simulink model "after_regulation"  (R2018a)
settings: Solver=VariableStepAuto  StartTime=0.0  StopTime=10.0  RelTol=1e-3
undefined symbols (not defined in the file or in its folder): sigbuilder_block
libraries: fuzblock x1
settings Model: Creator=root  LastModifiedBy=root

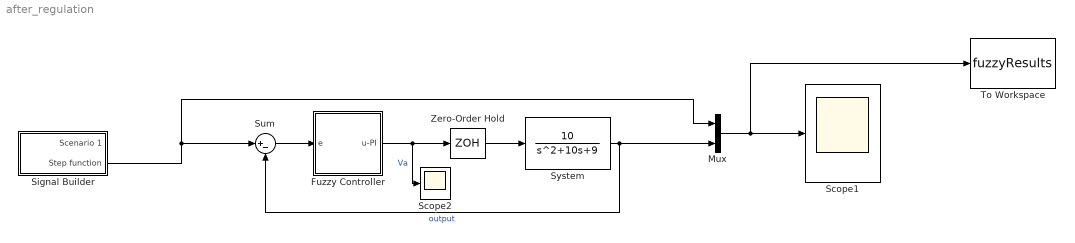
== system after_regulation ==
  Fuzzy Controller : Subsystem
  Mux : Mux  Inputs=2
  Scope1 : Scope
  Scope2 : Scope
  Signal Builder : Subsystem  Tag=STV Subsys  LoadFcn=sigbuilder_block('load');  StartFcn=sigbuilder_block('start');  StopFcn=sigbuilder_block('stop');  ClipboardFcn=sigbuilder_block('clipboard');  mask(Sigbuilder block){tuvar=[0:10]}
      mask help: Simulink:masks:SigbuilderBlock_MD
      mask init:
      | if ~strcmp(get_param(bdroot(gcbh),'SimulationStatus'),'stopped') tuvar = sigbuilder_block('maskInit'); end
      settings: CopyFcn=sigbuilder_block('copy');  DeleteFcn=sigbuilder_block('delete');  ModelCloseFcn=sigbuilder_block('modelClose');  PreSaveFcn=sigbuilder_block('preSave');  PauseFcn=sigbuilder_block('pause');  ContinueFcn=sigbuilder_block('continue');  NameChangeFcn=sigbuilder_block('namechange');  OpenFcn=sigbuilder_block('open',[225 75 550.5 393.75 ]);  CloseFcn=sigbuilder_block('close');
      mask Display: plot(0, 0, 100, 100,[2, 2, 32, 32, 2], [68, 8, 8, 68, 68],[32, 2], [38, 38], [32, 19, 2],[53, 60, 44], [32, 17, 17, 2],[16, 16, 31, 31]);txt = getActiveGroup(gcbh);text(2, 100, txt,'verticalAlignment', 'top');
  Sum : Sum  Inputs=|+-
  System : TransferFcn  Numerator=10  Denominator=[1 10 9]
  To Workspace : ToWorkspace  VariableName=fuzzyResults  SaveFormat=Timeseries  SampleTime=-1
  Zero-Order Hold : ZeroOrderHold  SampleTime=0.01
  wires:
  Zero-Order Hold/1 -> System/1
  System/1 -> Mux/2, Sum/2  "output"
  Fuzzy Controller/1(u-PI) -> Scope2/1, Zero-Order Hold/1  "Va"
  Signal Builder/2(Step function) -> Mux/1, Sum/1
  Sum/1 -> Fuzzy Controller/1(e)
  Mux/1 -> To Workspace/1, Scope1/1

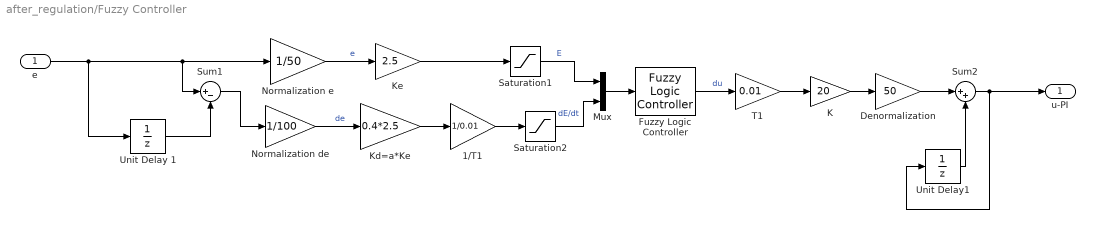
== system after_regulation/Fuzzy Controller ==
  e : Inport
  1/T1 : Gain  Gain=1/0.01
  Denormalization : Gain  Gain=50
  Fuzzy Logic Controller : fuzblock/Fuzzy Logic  Controller  FIS='satellite_8885'  OutputSampleNumber=101  DataType=single  FuzzifiedInputs=off  RuleFiringStrengths=off  RuleOutputs=off  AggregatedOutputs=off  SimulateUsing=Interpreted execution  OutOfRangeInputValueMessage=warning  NoRuleFiredMessage=warning  EmptyOutputFuzzySetMessage=warning
  K : Gain  Gain=20
  Kd=a*Ke : Gain  Gain=0.4*2.5
  Ke : Gain  Gain=2.5
  Mux : Mux  Inputs=2
  Normalization de : Gain  Gain=1/100
  Normalization e : Gain  Gain=1/50
  Saturation1 : Saturate  UpperLimit=1  LowerLimit=-1
  Saturation2 : Saturate  UpperLimit=1  LowerLimit=-1
  Sum1 : Sum  Inputs=|+-
  Sum2 : Sum  Inputs=|++
  T1 : Gain  Gain=0.01
  Unit Delay 1 : UnitDelay  SampleTime=-1
  Unit Delay1 : UnitDelay  SampleTime=-1
  u-PI : Outport
  wires:
  Normalization e/1 -> Ke/1  "e"
  Normalization de/1 -> Kd=a*Ke/1  "de"
  Saturation2/1 -> Mux/2  "dE/dt"
  e/1 -> Unit Delay 1/1, Sum1/1, Normalization e/1
  Unit Delay 1/1 -> Sum1/2
  Sum2/1 -> Unit Delay1/1, u-PI/1
  Saturation1/1 -> Mux/1  "E"
  Unit Delay1/1 -> Sum2/2
  Kd=a*Ke/1 -> 1/T1/1
  K/1 -> Denormalization/1
  Denormalization/1 -> Sum2/1
  Sum1/1 -> Normalization de/1
  Ke/1 -> Saturation1/1
  1/T1/1 -> Saturation2/1
  Mux/1 -> Fuzzy Logic Controller/1
  T1/1 -> K/1
  Fuzzy Logic Controller/1 -> T1/1  "du"

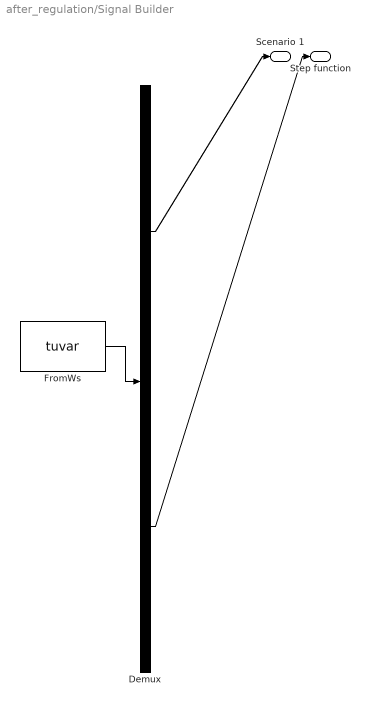
== system after_regulation/Signal Builder ==
  Demux : Demux  Tag=STV Demux  Outputs=2
  FromWs : FromWorkspace  Tag=STV FromWs  VariableName=tuvar  SampleTime=0
      SigBuilderData=|
      | common.afterFinalStr = 'Extrapolate'
      | common.sampleTime = 0
      | dataSet.timeRange = [0 30]
      | dataSet.name = 'Group 1'
      | sbobj.Groups.Name = 'Group 1'
      | sbobj.Groups.Signals(1).Name = 'Scenario 1'
      | sbobj.Groups.Signals(1).XData = [0 10 10 20 20 30]
      | sbobj.Groups.Signals(1).YData = [150 150 100 100 150 150]
      | sbobj.Groups.Signals(2).Name = 'Step function'
      | sbobj.Groups.Signals(2).XData = [0 30]
      | sbobj.Groups.Signals(2).YData = [50 50]
      | sbobj.Groups.TimeRange = [0 30]
  Scenario 1 : Outport  Tag=STV Outport
  Step function : Outport  Tag=STV Outport  Port=2
  wires:
  FromWs/1 -> Demux/1
  Demux/1 -> Scenario 1/1
  Demux/2 -> Step function/1
